simulink model "RightArmAgent"  (Simulink 6.5)
settings: Solver=ode45  SolverMode=SingleTasking  StartTime=0.0  StopTime=10.0  RelTol=1e-3  AbsTol=1e-6
settings Model: Creator=The MathWorks Inc.  LastModifiedBy=suarezjl  ExtModeTrigMode=oneshot  ExtModeArmWhenConnect=off  ExtModeAutoUpdateStatusClock=off
settings DataIOCC: LimitDataPoints=off  SignalLoggingName=logsOut
settings OptimizationCC: BooleanDataType=off  InlineInvariantSignals=on
settings DebuggingCC: CheckExecutionContextPreStartOutputMsg=on  CheckExecutionContextRuntimeOutputMsg=on  SolverPrmCheckMsg=none  MultiTaskDSMMsg=warning  MultiTaskCondExecSysMsg=none  IntegerOverflowMsg=none  StrictBusMsg=None
settings HardwareCC: TargetUnknown=on
settings ModelReferenceCC: UpdateModelReferenceTargets=IfOutOfDate
settings RTWCC: IncludeERTFirstTime=on

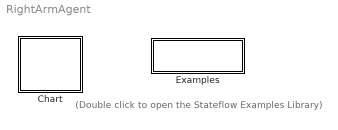
== system RightArmAgent ==
  note: (Double click to open the
      | Stateflow Examples Library)
  Chart : Stateflow chart
  Examples : Subsystem
      settings: OpenFcn=sf('Private','sf_examples')
      mask Display: disp('Examples')

== system RightArmAgent/Examples ==

== stateflow chart Chart ==
  state Homing Routine
    Hungerforce\RightReachDemo\RightArm\SampleIndPressure.Disable_ZMasking()
    Hungerforce\RightReachDemo\RightArm\HomingController.Initial()
    Hungerforce\RightReachDemo\RightArm\HomingController.ComputeHomingPressures()
    Hungerforce\RightReachDemo\RightArm\SampleIndPressure.HW_IO_6()
    Hungerforce\RightReachDemo\RightArm\StateMachine.Wait(50)
  state InitializeFunctions
    Hungerforce\RightReachDemo\RightArm\SampleIndPressure.Initialize()
    Hungerforce\RightReachDemo\RightArm\PIDNonLinCtrl.Initial()
    Hungerforce\RightReachDemo\RightArm\ForwardKinematics.Initialize()
    Hungerforce\RightReachDemo\RightArm\InverseKinematics.Initialize()
  state WriteHomeDesiredLogicalAngles
    Hungerforce\RightReachDemo\RightArm\SampleIndPressure.Enable_ZMasking()
    Hungerforce\RightReachDemo\RightArm\SampleIndPressure.WriteHomePositions()
  state LoadHomePosition
    Hungerforce\RightReachDemo\RightArm\SampleIndPressure.HW_IO_6()
    Hungerforce\RightReachDemo\RightArm\PIDNonLinCtrl.PID_NonLin_6Press()
    Hungerforce\RightReachDemo\RightArm\ForwardKinematics.ForwardKinematics()
    Hungerforce\RightReachDemo\RightArm\InverseKinematics.InverseKinematics()
  state PID_NonLinCtrlLoop
    Hungerforce\RightReachDemo\RightArm\Filter.FilterDesiredAngles()
    Hungerforce\RightReachDemo\RightArm\PIDNonLinCtrl.PID_NonLin_12Press()
    Hungerforce\RightReachDemo\RightArm\SampleIndPressure.HW_IO_12()
    Hungerforce\RightReachDemo\RightArm\PIDNonLinCtrl.Read_CurrentPressure()
    Hungerforce\RightReachDemo\RightArm\ForwardKinematics.ForwardKinematics()
    Hungerforce\RightReachDemo\RightArm\InverseKinematics.InverseKinematics()
    Hungerforce\RightReachDemo\RightArm\StateMachine.Wait(50)
  state Fire event to start Trajectory Generation in Hungerforce
    \\Hungerforce\RightReachDemo\RightTrajectoryAgent\StateMachine.LoadSM()
    \\Hungerforce\RightReachDemo\RightTrajectoryAgent\StateMachine.Start()
  (default) -> InitializeFunctions : Start
  Homing Routine -> Homing Routine [order 1] : Default
  InitializeFunctions -> Homing Routine : Always
  WriteHomeDesiredLogicalAngles -> LoadHomePosition : Always
  LoadHomePosition -> Fire event to start Trajectory Generation in Hungerforce : Always
  Homing Routine -> WriteHomeDesiredLogicalAngles [order 2] : Signal="Go to next state"
  PID_NonLinCtrlLoop -> PID_NonLinCtrlLoop : Default
  Fire event to start Trajectory Generation in Hungerforce -> PID_NonLinCtrlLoop : Always
